simulink model "connect_pend"  (R2019b)
settings: Solver=VariableStepAuto  StartTime=0.0  StopTime=10.0  RelTol=1e-3
values from neighbouring files (symbols this model uses):
  dampener = 100    [anujay_single_pendulum_same.m]    (also in connect_pend.m; connect_pend_runner.m = 300; double_pend_setup.m = [50, 0; 0, 50])
  g = 9.81    [G.m]    (also in connect_pend_runner.m = -9.81; run.m; single_pend_runner.m = -9.81)
  Kd = 50    [anujay_single_pendulum_same.m]    (also in connect_pend_runner.m = 10; double_pend_setup.m = [50,0;0,50]; single_pend_runner.m = 500)
  Kp = 500    [single_pend_runner.m]
  l = [ 1.0, 1.5]    [double_pend_setup.m]    (also in run.m = 1)
  l1 = 1.0    (= 1)    [connect_pend.m]    (also in connect_pend_runner.m)
  m1 = 1.0    (= 1)    [connect_pend.m]    (also in connect_pend_runner.m)
  spring = 100    [anujay_single_pendulum_same.m]    (also in connect_pend.m; connect_pend_runner.m = 300; double_pend_setup.m = [50, 0; 0, 50])
undefined symbols (not defined in the file or in its folder): m
settings Model: Creator=nathanielgoldfarb  LastModifiedBy=nathanielgoldfarb

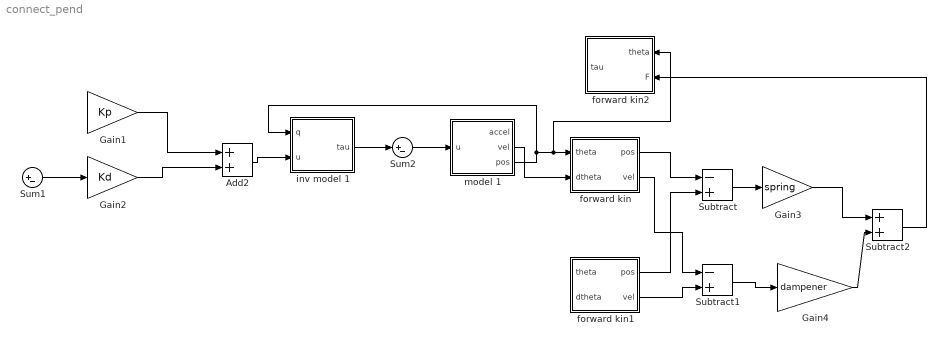
== system connect_pend ==
  Add2 : Sum
  Gain1 : Gain  Gain=Kp
  Gain2 : Gain  Gain=Kd
  Gain3 : Gain  Gain=spring
  Gain4 : Gain  Gain=dampener
  Subtract : Sum  Inputs=-+
  Subtract1 : Sum  Inputs=-+
  Subtract2 : Sum
  Sum1 : Sum  Inputs=|+-
  Sum2 : Sum  Inputs=|+-
  forward kin : Subsystem
  forward kin1 : Subsystem
  forward kin2 : Subsystem
  inv model 1 : Subsystem
  model 1 : Subsystem
  wires:
  Sum1/1 -> Gain2/1
  Sum2/1 -> model 1/1("u ")
  Add2/1 -> inv model 1/2("u ")
  inv model 1/1("tau ") -> Sum2/1
  Gain1/1 -> Add2/1
  Gain2/1 -> Add2/2
  model 1/3(pos) -> inv model 1/1(q), forward kin2/1("theta "), forward kin/1("theta ")
  model 1/2(vel) -> forward kin/2("dtheta ")
  forward kin1/1(pos) -> Subtract/2
  forward kin/1(pos) -> Subtract/1
  forward kin1/2(vel) -> Subtract1/2
  forward kin/2(vel) -> Subtract1/1
  Subtract/1 -> Gain3/1
  Subtract1/1 -> Gain4/1
  Gain3/1 -> Subtract2/1
  Gain4/1 -> Subtract2/2
  Subtract2/1 -> forward kin2/2(F)

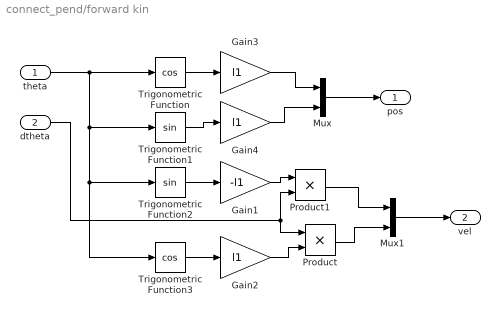
== system connect_pend/forward kin ==
  "theta " : Inport
  "dtheta " : Inport  Port=2
  Gain1 : Gain  Gain=-l1
  Gain2 : Gain  Gain=l1
  Gain3 : Gain  Gain=l1
  Gain4 : Gain  Gain=l1
  Mux : Mux  Inputs=2
  Mux1 : Mux  Inputs=2
  Product : Product
  Product1 : Product
  Trigonometric Function : Trigonometry  Operator=cos
  Trigonometric Function1 : Trigonometry
  Trigonometric Function2 : Trigonometry
  Trigonometric Function3 : Trigonometry  Operator=cos
  pos : Outport
  vel : Outport  Port=2
  wires:
  "theta "/1 -> Trigonometric Function3/1, Trigonometric Function2/1, Trigonometric Function1/1, Trigonometric Function/1
  Gain4/1 -> Mux/2
  Trigonometric Function/1 -> Gain3/1
  Gain3/1 -> Mux/1
  Trigonometric Function1/1 -> Gain4/1
  Trigonometric Function3/1 -> Gain2/1
  Trigonometric Function2/1 -> Gain1/1
  Gain1/1 -> Product1/1
  "dtheta "/1 -> Product1/2, Product/1
  Gain2/1 -> Product/2
  Product1/1 -> Mux1/1
  Product/1 -> Mux1/2
  Mux/1 -> pos/1
  Mux1/1 -> vel/1

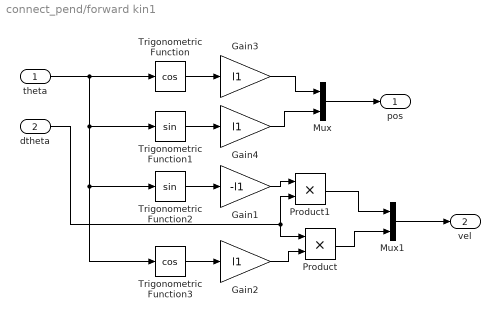
== system connect_pend/forward kin1 ==
  "theta " : Inport
  "dtheta " : Inport  Port=2
  Gain1 : Gain  Gain=-l1
  Gain2 : Gain  Gain=l1
  Gain3 : Gain  Gain=l1
  Gain4 : Gain  Gain=l1
  Mux : Mux  Inputs=2
  Mux1 : Mux  Inputs=2
  Product : Product
  Product1 : Product
  Trigonometric Function : Trigonometry  Operator=cos
  Trigonometric Function1 : Trigonometry
  Trigonometric Function2 : Trigonometry
  Trigonometric Function3 : Trigonometry  Operator=cos
  pos : Outport
  vel : Outport  Port=2
  wires:
  "theta "/1 -> Trigonometric Function3/1, Trigonometric Function2/1, Trigonometric Function1/1, Trigonometric Function/1
  Gain4/1 -> Mux/2
  Trigonometric Function/1 -> Gain3/1
  Gain3/1 -> Mux/1
  Trigonometric Function1/1 -> Gain4/1
  Trigonometric Function3/1 -> Gain2/1
  Trigonometric Function2/1 -> Gain1/1
  Gain1/1 -> Product1/1
  "dtheta "/1 -> Product1/2, Product/1
  Gain2/1 -> Product/2
  Product1/1 -> Mux1/1
  Product/1 -> Mux1/2
  Mux/1 -> pos/1
  Mux1/1 -> vel/1

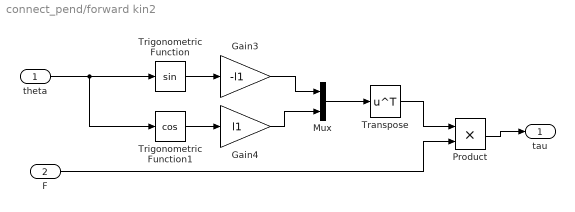
== system connect_pend/forward kin2 ==
  "theta " : Inport
  F : Inport  Port=2
  Gain3 : Gain  Gain=-l1
  Gain4 : Gain  Gain=l1
  Mux : Mux  Inputs=2
  Product : Product
  Transpose : Math  Operator=transpose  SignedPower=off  SaturateOnIntegerOverflow=on
  Trigonometric Function : Trigonometry
  Trigonometric Function1 : Trigonometry  Operator=cos
  "tau " : Outport
  wires:
  "theta "/1 -> Trigonometric Function1/1, Trigonometric Function/1
  Gain4/1 -> Mux/2
  Trigonometric Function/1 -> Gain3/1
  Gain3/1 -> Mux/1
  Trigonometric Function1/1 -> Gain4/1
  Mux/1 -> Transpose/1
  Transpose/1 -> Product/1
  F/1 -> Product/2
  Product/1 -> "tau "/1

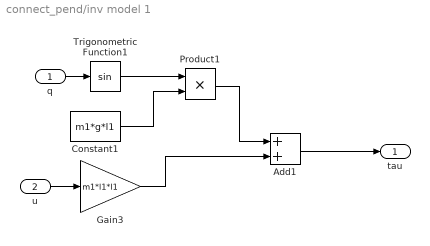
== system connect_pend/inv model 1 ==
  q : Inport
  "u " : Inport  Port=2
  Add1 : Sum
  Constant1 : Constant  Value=m1*g*l1
  Gain3 : Gain  Gain=m1*l1*l1
  Product1 : Product
  Trigonometric Function1 : Trigonometry
  "tau " : Outport
  wires:
  Product1/1 -> Add1/1
  Constant1/1 -> Product1/2
  Add1/1 -> "tau "/1
  Gain3/1 -> Add1/2
  "u "/1 -> Gain3/1
  Trigonometric Function1/1 -> Product1/1
  q/1 -> Trigonometric Function1/1

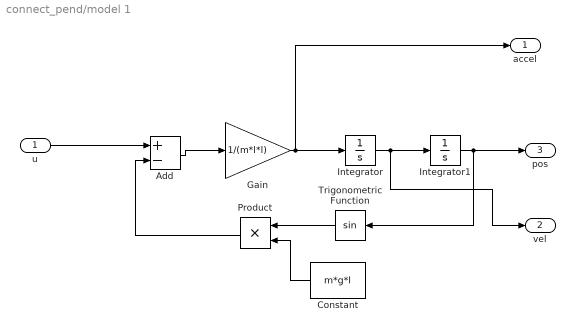
== system connect_pend/model 1 ==
  "u " : Inport
  Add : Sum  Inputs=+-
  Constant : Constant  Value=m*g*l
  Gain : Gain  Gain=1/(m*l*l)
  Integrator : Integrator
  Integrator1 : Integrator  InitialCondition=-pi
  Product : Product
  Trigonometric Function : Trigonometry
  accel : Outport
  vel : Outport  Port=2
  pos : Outport  Port=3
  wires:
  Integrator1/1 -> pos/1, Trigonometric Function/1
  "u "/1 -> Add/1
  Constant/1 -> Product/2
  Add/1 -> Gain/1
  Trigonometric Function/1 -> Product/1
  Product/1 -> Add/2
  Gain/1 -> accel/1, Integrator/1
  Integrator/1 -> vel/1, Integrator1/1
